simulink model "Ac_ac_converters"  (R2024a)
settings: Solver=VariableStepAuto  StartTime=0.0  StopTime=15  RelTol=1e-3
undefined symbols (not defined in the file or in its folder): D1, lagging, pulse
libraries: spsThyristorLib x6, spsThreePhaseVIMeasurementLib x2, spsThreePhaseBreakerLib x2, spsPLL3phLib x1, spsPulseGeneratorThyristor12PulseLib x1
settings Model: Creator=gshma  LastModifiedBy=gshma

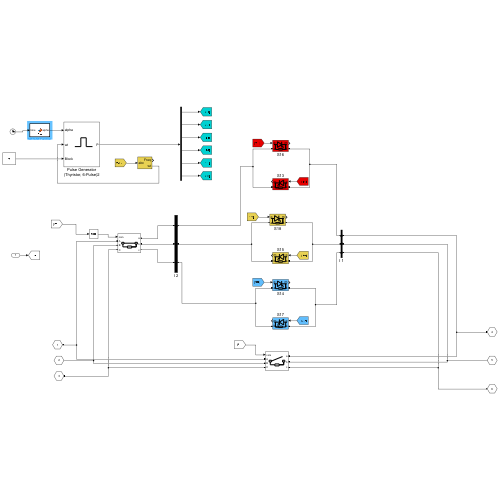
[thumbnail: Simulink's stored preview of the top-level diagram]
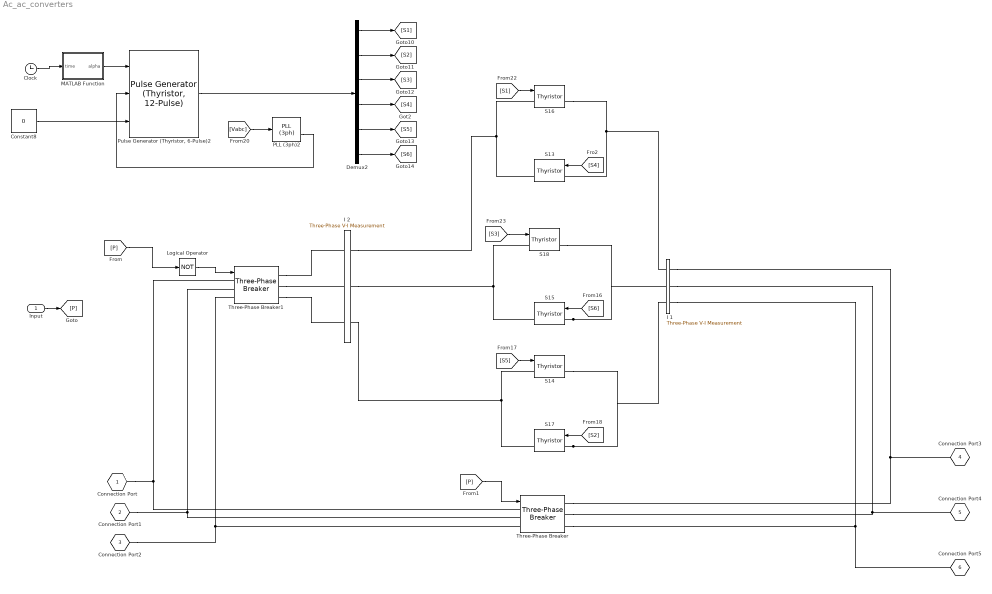
== system Ac_ac_converters ==
  Input : Inport
  Clock : Clock
  Constant8 : Constant  Value=0
  Demux2 : Demux  Outputs=6
  I 1 : spsThreePhaseVIMeasurementLib/Three-Phase V-I Measurement  VoltageMeasurement=phase-to-phase  SetLabelV=on  LabelV=Vabc1  Vpu=off  VpuLL=off  CurrentMeasurement=yes  SetLabelI=on  LabelI=Iabc1  Ipu=off  Pbase=100e6  Vbase=500e3  OutputType=Complex  PhasorSimulation=off  PSBequivalent=0
  I 2 : spsThreePhaseVIMeasurementLib/Three-Phase V-I Measurement  VoltageMeasurement=phase-to-ground  SetLabelV=on  LabelV=Vabc  Vpu=off  VpuLL=off  CurrentMeasurement=yes  SetLabelI=on  LabelI=Iab  Ipu=off  Pbase=100e6  Vbase=500e3  OutputType=Complex  PhasorSimulation=off  PSBequivalent=0
  Logical Operator : Logic  Operator=NOT  AllPortsSameDT=off  OutDataTypeStr=boolean
  MATLAB Function : MATLAB Function  TreatAsAtomicUnit=on
  PLL (3ph)2 : spsPLL3phLib/PLL (3ph)  Fmin=45  Par_Init=[0, 50]  ParK=[180, 3200, 1]  TcD=1e-4  MaxRateChangeFreq=12  FilterCutOffFreq=25  Ts=0  AGC=on
  "Pulse Generator (Thyristor, 6-Pulse)2" : spsPulseGeneratorThyristor12PulseLib/Pulse Generator (Thyristor, 12-Pulse)  GenType=6-pulse  Delta=D1 (lagging)  pwidth=50  Double_Pulse=on  Ts=0
      settings: LibrarySourceBlock=|
      | sps_lib/Power Electronics/Power Electronics Control/Pulse Generator
      | (Thyristor, 12-Pulse)
  S{13..18} (6 alike) : spsThyristorLib/Thyristor  Ron=0.001  Lon=0  Vf=0.8  IC=0  Rs=500  Cs=250e-9  Measurements=on
  Three-Phase Breaker : spsThreePhaseBreakerLib/Three-Phase Breaker  InitialState=open  SwitchA=on  SwitchB=on  SwitchC=on  SwitchTimes="[1/60  5/60]"  External=on  BreakerResistance=0.01  SnubberResistance=1e6  SnubberCapacitance=inf  Measurements=None
  Three-Phase Breaker1 : spsThreePhaseBreakerLib/Three-Phase Breaker  InitialState=closed  SwitchA=on  SwitchB=on  SwitchC=on  SwitchTimes="[1/60  5/60]"  External=on  BreakerResistance=0.01  SnubberResistance=1e6  SnubberCapacitance=inf  Measurements=None
  Connection Port : PMIOPort  Tag=simrfV2util1/Connection Port  Side=Left
  Connection Port1 : PMIOPort  Tag=simrfV2util1/Connection Port  Port=2  Side=Left
  Connection Port2 : PMIOPort  Tag=simrfV2util1/Connection Port  Port=3  Side=Left
  Connection Port3 : PMIOPort  Tag=simrfV2util1/Connection Port  Port=4  Side=Right
  Connection Port4 : PMIOPort  Tag=simrfV2util1/Connection Port  Port=5  Side=Right
  Connection Port5 : PMIOPort  Tag=simrfV2util1/Connection Port  Port=6  Side=Right
  wires:
  Demux2/3 -> [S3]
  [S5] -> S14/1
  PLL (3ph)2/2 -> "Pulse Generator (Thyristor, 6-Pulse)2"/2
  [S4] -> S13/1
  Demux2/1 -> [S1]
  Demux2/4 -> [S4]
  [Vabc] -> PLL (3ph)2/1
  [S2] -> S17/1
  Demux2/2 -> [S2]
  [S1] -> S16/1
  [S3] -> S18/1
  Demux2/6 -> [S6]
  "Pulse Generator (Thyristor, 6-Pulse)2"/1 -> Demux2/1
  [S6] -> S15/1
  Constant8/1 -> "Pulse Generator (Thyristor, 6-Pulse)2"/3
  Demux2/5 -> [S5]
  Clock/1 -> MATLAB Function/1(time)
  MATLAB Function/1(alpha) -> "Pulse Generator (Thyristor, 6-Pulse)2"/1
  Input/1 -> [P]
  Logical Operator/1 -> Three-Phase Breaker1/1
  [P] -> Logical Operator/1
  [P] -> Three-Phase Breaker/1
  connections:
  S14/LConn1 -- I 2/RConn3 -- S17/RConn1
  S13/RConn1 -- S16/LConn1 -- I 2/RConn1
  I 1/LConn1 -- S16/RConn1 -- S13/LConn1
  S18/LConn1 -- S15/RConn1 -- I 2/RConn2
  S17/LConn1 -- S14/RConn1 -- I 1/LConn3
  S15/LConn1 -- S18/RConn1 -- I 1/LConn2
  Connection Port/RConn1 -- Three-Phase Breaker1/LConn1 -- Three-Phase Breaker/LConn1
  Connection Port1/RConn1 -- Three-Phase Breaker1/LConn2 -- Three-Phase Breaker/LConn2
  Connection Port2/RConn1 -- Three-Phase Breaker1/LConn3 -- Three-Phase Breaker/LConn3
  Three-Phase Breaker/RConn1 -- I 1/RConn1 -- Connection Port3/RConn1
  Three-Phase Breaker/RConn2 -- I 1/RConn2 -- Connection Port4/RConn1
  Three-Phase Breaker/RConn3 -- Connection Port5/RConn1 -- I 1/RConn3
  Three-Phase Breaker1/RConn1 -- I 2/LConn1
  Three-Phase Breaker1/RConn2 -- I 2/LConn2
  Three-Phase Breaker1/RConn3 -- I 2/LConn3

== matlab function Ac_ac_converters/MATLAB Function ==
  data: time input; alpha output
function alpha = fcn(time)
    if time < 2
        alpha = 100;
    elseif time >= 2 && time < 3.5
        alpha = 90;
    elseif time >= 3.5 && time < 4.5
        alpha = 60;
    elseif time >= 4.5 && time < 6
        alpha = 40;
    elseif time >= 6 && time < 7.5
        alpha = 30;
    elseif time >= 7.5 && time < 8
        alpha = 10;
    else
        alpha = 0;
    end
end
